simulink model "Lab08_Simulink"  (R2020b)
settings: Solver=VariableStepAuto  StartTime=0.0  StopTime=10.0  RelTol=1e-3
PreLoadFcn:
  | fs = 1e3; % frecuencia de muestreo
  | Ts = 1/fs; % tiempo de muestra
  | Tb = 0.1; % tiempo de bit
  | Tc = 0.01; % tiempo de chip
  | frameSize = 1000; % tama~no de cada marco en bloques de origen
InitFcn:
  | fs = 1e3;% frecuencia de muestreo
  | Ts = 1/fs; % tiempo de muestra
  | Tb = 0.1; % tiempo de bit
  | Tc = 0.01; % tiempo de chip
  | frameSize = 1000; % tama~no de cada marco en bloques de origen
libraries: commfilt2 x4, commchan3 x1, commdigbbndpm3 x1, commrandsrc3 x1
settings Model: Creator=Diego  LastModifiedBy=Diego

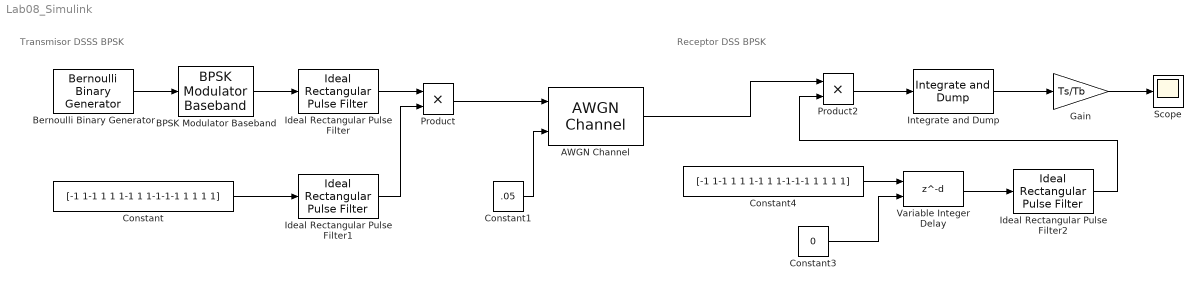
== system Lab08_Simulink ==
  note: Receptor DSS BPSK
  note: Transmisor DSSS BPSK
  AWGN Channel : commchan3/AWGN Channel  InputProcessing=Columns as channels (frame based)  seed=var  noiseMode=Variance from port  EbNodB=10  EsNodB=10  SNRdB=10  bitsPerSym=1  Ps=1  Tsym=1  variance=1
  BPSK Modulator Baseband : commdigbbndpm3/BPSK Modulator Baseband  Ph=0  outDtype=double  outWordLen=16  outUDDataType=sfix(16)  outFracLenMode=Best precision  outFracLen=15  outDataTypeStr=double  outLastDataTypeStr=double
  Bernoulli Binary Generator : commrandsrc3/Bernoulli Binary Generator  ProbabilityOfZero=0.5  SeedSource=Auto  Seed=0  SampleTime=1  SamplesPerFrame=1  OutputDataType=double  SimulateUsing=Interpreted execution
  Constant : Constant  Value=[-1 1-1 1 1 1-1 1 1-1-1-1 1 1 1 1]
  Constant1 : Constant  Value=.05
  Constant3 : Constant  Value=0
  Constant4 : Constant  Value=[-1 1-1 1 1 1-1 1 1-1-1-1 1 1 1 1]
  Gain : Gain  Gain=Ts/Tb
  Ideal Rectangular Pulse Filter : commfilt2/Ideal Rectangular Pulse Filter  pulseLen=1  pulseDelay=0  InputProcessing=Columns as channels (frame based)  RateOptions=Enforce single-rate processing  sampMode=Mute  normCheck=off  normMode=Sum of samples  filterGain=1  saveAsFlag=0  roundingMode=Floor  overflowMode=off  firstCoeffDataTypeStr=Inherit: Same word length as input  firstCoeffMin=[]  firstCoeffMax=[]  firstCoeffLastDataTypeStr=Inherit: Same word length as input  outputDataTypeStr=Inherit: Same as accumulator  outputMin=[]  outputMax=[]  outputLastDataTypeStr=Inherit: Same as accumulator
      settings: SourceProductBaseCode=CM
  Ideal Rectangular Pulse Filter1 : commfilt2/Ideal Rectangular Pulse Filter  pulseLen=1  pulseDelay=0  InputProcessing=Columns as channels (frame based)  RateOptions=Allow multirate processing  sampMode=Mute  normCheck=off  normMode=Sum of samples  filterGain=1  saveAsFlag=0  roundingMode=Floor  overflowMode=off  firstCoeffDataTypeStr=Inherit: Same word length as input  firstCoeffMin=[]  firstCoeffMax=[]  firstCoeffLastDataTypeStr=Inherit: Same word length as input  outputDataTypeStr=Inherit: Same as accumulator  outputMin=[]  outputMax=[]  outputLastDataTypeStr=Inherit: Same as accumulator
      settings: SourceProductBaseCode=CM
  Ideal Rectangular Pulse Filter2 : commfilt2/Ideal Rectangular Pulse Filter  pulseLen=1  pulseDelay=0  InputProcessing=Columns as channels (frame based)  RateOptions=Enforce single-rate processing  sampMode=Mute  normCheck=off  normMode=Sum of samples  filterGain=1  saveAsFlag=0  roundingMode=Floor  overflowMode=off  firstCoeffDataTypeStr=Inherit: Same word length as input  firstCoeffMin=[]  firstCoeffMax=[]  firstCoeffLastDataTypeStr=Inherit: Same word length as input  outputDataTypeStr=Inherit: Same as accumulator  outputMin=[]  outputMax=[]  outputLastDataTypeStr=Inherit: Same as accumulator
      settings: SourceProductBaseCode=CM
  Integrate and Dump : commfilt2/Integrate and Dump  obssamples=8  offsetsamples=0  nodump=off  roundingMode=Floor  overflowMode=off  outputDataTypeStr=Inherit: Same as accumulator  outputLastDataTypeStr=Inherit: Same as accumulator
  Product : Product  InputSameDT=on
  Product2 : Product
  Scope : Scope
  Variable Integer Delay : Delay  DelayLengthSource=Input port
      settings: InputPortMap=u0,p1
  wires:
  Bernoulli Binary Generator/1 -> BPSK Modulator Baseband/1
  BPSK Modulator Baseband/1 -> Ideal Rectangular Pulse Filter/1
  Ideal Rectangular Pulse Filter/1 -> Product/1
  Constant/1 -> Ideal Rectangular Pulse Filter1/1
  Ideal Rectangular Pulse Filter1/1 -> Product/2
  Product2/1 -> Integrate and Dump/1
  Ideal Rectangular Pulse Filter2/1 -> Product2/2
  Variable Integer Delay/1 -> Ideal Rectangular Pulse Filter2/1
  Constant3/1 -> Variable Integer Delay/2
  Product/1 -> AWGN Channel/1
  Constant1/1 -> AWGN Channel/2
  AWGN Channel/1 -> Product2/1
  Integrate and Dump/1 -> Gain/1
  Gain/1 -> Scope/1
  Constant4/1 -> Variable Integer Delay/1
